simulink model "launcher_dir"  (R2019a)
settings: Solver=ode45  StartTime=0.0  StopTime=5  RelTol=1e-3
libraries: fuzblock x1
settings Model: Creator=hlf  LastModifiedBy=83621
settings DataIOCC: SaveFormat=StructureWithTime
settings OptimizationCC: LifeSpan=inf
settings DebuggingCC: SFExecutionAtInitializationDiag=none  ArithmeticOperatorsInVariantConditions=warning
settings HardwareCC: ProdBitPerSizeT=32  ProdBitPerPtrDiffT=32  ProdWordSize=32  ProdHWDeviceType=Specified
settings CodeAppCC: StateflowObjectComments=on

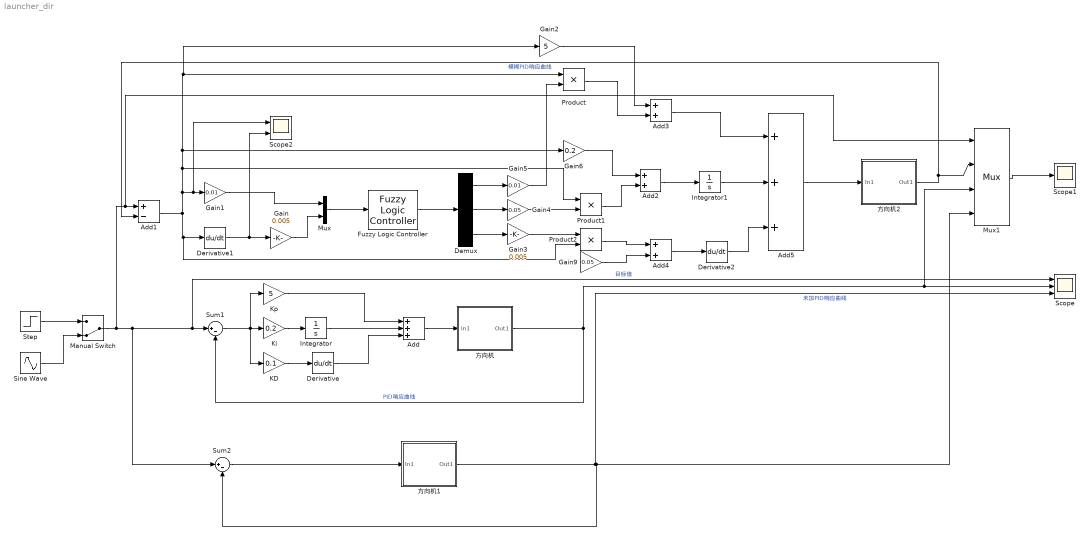
== system launcher_dir ==
  Add : Sum  Inputs=+++
  Add1 : Sum  Inputs=+-
  Add2 : Sum
  Add3 : Sum
  Add4 : Sum
  Add5 : Sum  Inputs=+++
  Demux : Demux  Outputs=3
  Derivative : Derivative
  Derivative1 : Derivative
  Derivative2 : Derivative
  Fuzzy Logic Controller : fuzblock/Fuzzy Logic  Controller  FIS='Fuzzy_PID.fis'  OutputSampleNumber=101  DataType=double  FuzzifiedInputs=off  RuleFiringStrengths=off  RuleOutputs=off  AggregatedOutputs=off  SimulateUsing=Interpreted execution  OutOfRangeInputValueMessage=warning  NoRuleFiredMessage=warning  EmptyOutputFuzzySetMessage=warning
  Gain : Gain  Gain=0.005
  Gain1 : Gain  Gain=0.01
  Gain2 : Gain  Gain=5
  Gain3 : Gain  Gain=0.005
  Gain4 : Gain  Gain=0.05
  Gain5 : Gain  Gain=0.01
  Gain6 : Gain  Gain=0.2
  Gain9 : Gain  Gain=0.05
  Integrator : Integrator
  Integrator1 : Integrator
  KD : Gain  Gain=0.1
  "Ki " : Gain  Gain=0.2
  Kp : Gain  Gain=5
  Manual Switch : ManualSwitch  CurrentSetting=0
  Mux : Mux  Inputs=2
  Mux1 : Mux
  Product : Product
  Product1 : Product
  Product2 : Product
  Scope : Scope  NumInputPorts=3
  Scope1 : Scope
  Scope2 : Scope  NumInputPorts=2
  Sine Wave : Sin  Frequency=2  SampleTime=0
  Step : Step  Time=0  SampleTime=0
  Sum1 : Sum  Inputs=|+-
  Sum2 : Sum  Inputs=|+-
  方向机 : Subsystem
  方向机1 : Subsystem
  方向机2 : Subsystem
  wires:
  方向机/1(Out1) -> Sum1/2, Mux1/3, Scope/2  "PID响应曲线"
  Sum1/1 -> KD/1, Kp/1, "Ki "/1
  Manual Switch/1 -> Mux1/1, Add1/1, Sum2/1, Scope/1, Sum1/1  "目标值"
  Step/1 -> Manual Switch/1
  Sine Wave/1 -> Manual Switch/2
  "Ki "/1 -> Integrator/1
  KD/1 -> Derivative/1
  Integrator/1 -> Add/2
  Kp/1 -> Add/1
  Derivative/1 -> Add/3
  Add/1 -> 方向机/1(In1)
  Sum2/1 -> 方向机1/1(In1)
  方向机1/1(Out1) -> Mux1/4, Sum2/2, Scope/3  "未加PID响应曲线"
  Derivative1/1 -> Scope2/2, Gain/1
  Gain1/1 -> Mux/1
  Gain/1 -> Mux/2
  Mux/1 -> Fuzzy Logic Controller/1
  Fuzzy Logic Controller/1 -> Demux/1
  Demux/1 -> Gain5/1
  Demux/2 -> Gain4/1
  Demux/3 -> Gain3/1
  Add1/1 -> Scope2/1, Gain1/1, Product1/1, Gain2/1, Product/1, Gain6/1, Product2/2, Derivative1/1
  Gain5/1 -> Product/2
  Gain4/1 -> Product1/2
  Product1/1 -> Add2/2
  Gain6/1 -> Add2/1
  Product/1 -> Add3/2
  Gain2/1 -> Add3/1
  Add2/1 -> Integrator1/1
  Gain3/1 -> Product2/1
  Product2/1 -> Add4/1
  Gain9/1 -> Add4/2
  Add4/1 -> Derivative2/1
  Add3/1 -> Add5/1
  Integrator1/1 -> Add5/2
  Derivative2/1 -> Add5/3
  Add5/1 -> 方向机2/1(In1)
  Mux1/1 -> Scope1/1
  方向机2/1(Out1) -> Add1/2, Mux1/2  "模糊PID响应曲线"

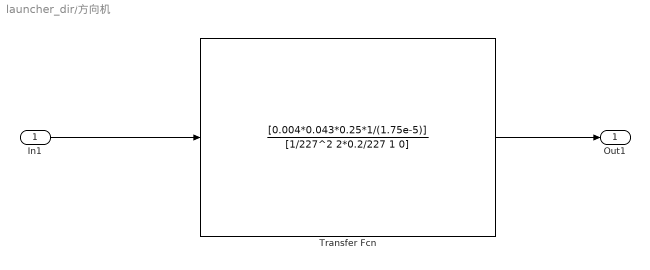
== system launcher_dir/方向机 ==
  In1 : Inport
  Transfer Fcn : TransferFcn  Numerator=[0.004*0.043*0.25*1/(1.75e-5)]  Denominator=[1/227^2 2*0.2/227 1 0]
  Out1 : Outport
  wires:
  Transfer Fcn/1 -> Out1/1
  In1/1 -> Transfer Fcn/1

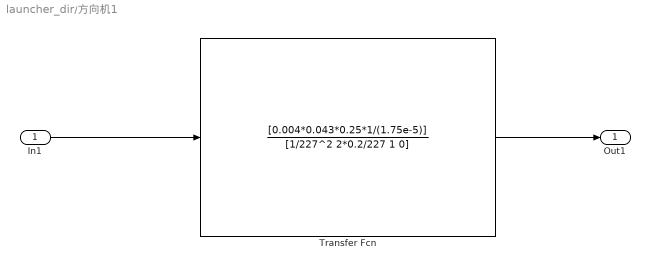
== system launcher_dir/方向机1 ==
  In1 : Inport
  Transfer Fcn : TransferFcn  Numerator=[0.004*0.043*0.25*1/(1.75e-5)]  Denominator=[1/227^2 2*0.2/227 1 0]
  Out1 : Outport
  wires:
  In1/1 -> Transfer Fcn/1
  Transfer Fcn/1 -> Out1/1

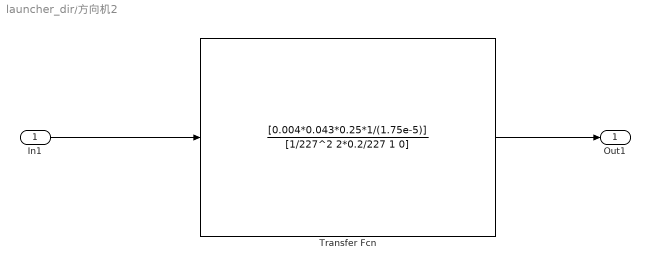
== system launcher_dir/方向机2 ==
  In1 : Inport
  Transfer Fcn : TransferFcn  Numerator=[0.004*0.043*0.25*1/(1.75e-5)]  Denominator=[1/227^2 2*0.2/227 1 0]
  Out1 : Outport
  wires:
  Transfer Fcn/1 -> Out1/1
  In1/1 -> Transfer Fcn/1
